simulink model "week4_4_final_cruise_control"  (R2025b)
settings: Solver=VariableStepAuto  StartTime=0.0  StopTime=100  MaxStep=0.01  RelTol=1e-3
undefined symbols (not defined in the file): A_front, Cd, Cr, g, m, rho, v0
libraries: slpidlib x1
settings Model: Creator=legob  LastModifiedBy=legob

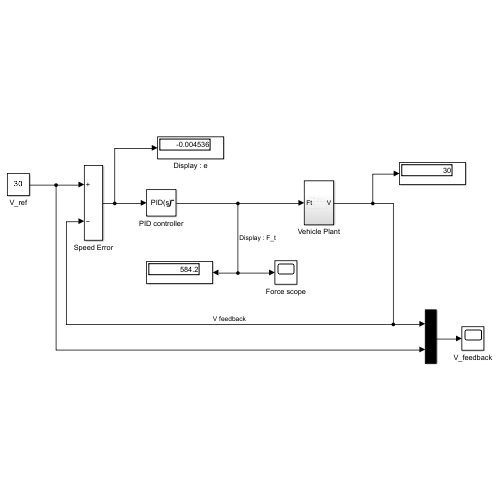
[thumbnail: Simulink's stored preview of the top-level diagram]
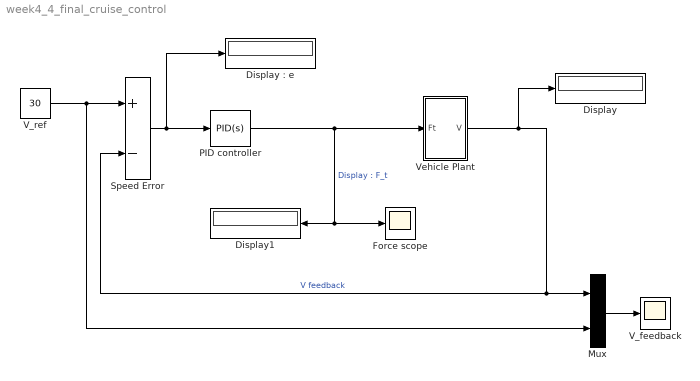
== system week4_4_final_cruise_control ==
  Display : Display
  "Display : e" : Display
  Display1 : Display
  Force scope : Scope
      settings: ActiveDisplayYMinimum=-292.64351118443733  ActiveDisplayYMaximum=5182.92090492779
  Mux : Mux  Inputs=2
  PID controller : slpidlib/PID Controller  Controller=PID  Form=Parallel  TimeDomain=Continuous-time  UseExternalTs=off  SampleTime=-1  IntegratorMethod=Forward Euler  FilterMethod=Forward Euler  ControllerParametersSource=internal  P=500  I=25  UseKiTs=off  D=500  UseExternalDerivativeSource=off  N=100  UseFilter=on  TunerSelectOption=Transfer Function Based (PID Tuner App)  InitialConditionSource=internal  InitialConditionForIntegrator=0  InitialConditionForFilter=0  DifferentiatorICPrevScaledInput=0  ExternalReset=none  TrackingMode=off  Kt=1  LimitOutput=on  SatLimitsSource=internal  UpperSaturationLimit=4000  LowerSaturationLimit=0  LinearizeAsGain=on  AntiWindupMode=clamping  Kb=1  LimitIntegrator=off  UpperIntegratorSaturationLimit=inf  LowerIntegratorSaturationLimit=-inf  POutMin=[]  POutMax=[]  IOutMin=[]  IOutMax=[]  DOutMin=[]  DOutMax=[]  NOutMin=[]  NOutMax=[]  SumOutMin=[]  SumOutMax=[]  SaturationOutMin=[]  SaturationOutMax=[]  PParamMin=[]  PParamMax=[]  IParamMin=[]  IParamMax=[]  DParamMin=[]  DParamMax=[]  NParamMin=[]  NParamMax=[]  KbParamMin=[]  KbParamMax=[]  KtParamMin=[]  KtParamMax=[]  KbOutMin=[]  KbOutMax=[]  KtOutMin=[]  KtOutMax=[]  IntegratorOutMin=[]  IntegratorOutMax=[]  FilterOutMin=[]  FilterOutMax=[]  SumI1OutMin=[]  SumI1OutMax=[]  SumI2OutMin=[]  SumI2OutMax=[]  SumI3OutMin=[]  SumI3OutMax=[]  SumI4OutMin=[]  SumI4OutMax=[]  SumDOutMin=[]  SumDOutMax=[]  DifferentiatorOutMin=[]  DifferentiatorOutMax=[]  FilterDiffOutCoefMin=[]  FilterDiffOutCoefMax=[]  ReciprocalOutMin=[]  ReciprocalOutMax=[]  SumDenOutMin=[]  SumDenOutMax=[]  SumNumOutMin=[]  SumNumOutMax=[]  DivideOutMin=[]  DivideOutMax=[]  UdiffTsProdOutMin=[]  UdiffTsProdOutMax=[]  NTsProdOutMin=[]  NTsProdOutMax=[]  UintegralTsProdOutMin=[]  UintegralTsProdOutMax=[]  UngainTsProdOutMin=[]  UngainTsProdOutMax=[]  ClampingZeroOutDataTypeStr=Inherit: Inherit via back propagation  ClampingZeroOutMin=[]  ClampingZeroOutMax=[]  FilterDenConstantOutDataTypeStr=Inherit: Inherit via back propagation  FilterDenConstantOutMin=[]  FilterDenConstantOutMax=[]  PCopyOutDataTypeStr=Inherit: Inherit via back propagation  PCopyOutMin=[]  PCopyOutMax=[]  NCopyOutDataTypeStr=Inherit: Inherit via back propagation  NCopyOutMin=[]  NCopyOutMax=[]  IntegratorContinuousStateAttributes=''  IntegratorStateMustResolveToSignalObject=off  IntegratorRTWStateStorageClass=Auto  FilterContinuousStateAttributes=''  FilterStateMustResolveToSignalObject=off  FilterRTWStateStorageClass=Auto  ParallelPVariant=InternalParameters  IdealPVariant=Disabled  IVariant=InternalParameters  DVariant=InternalParameters  IntegratorVariant=Continuous  SatVariant=Enabled  AWVariant=ContClampingParallel  PCopyVariant=Disabled  TRVariant=Disabled  FdbkBlocksVariant=Forward  IdealPFdbkVariant=Disabled  SatFdbkVariant=Disabled  DerivativeFilterVariant=ContFilter  NVariant=InternalParameters  NCopyVariant=Disabled  FilterICVariant=InternalICsFilter  IntegratorICVariant=InternalICs  ExternalResetVariant=Disabled  TRSumVariant=Passthrough  SumFdbkVariant=Disabled  SumVariant=Sum_PID  TsampFilterVariant=InternalTs  TsampNgainVariant=Passthrough  TsampIntegralVariant=Disabled_SignalSpec  ExternalSaturationOutDataTypeStr=Inherit: Same as second input  DerivativeSourceVariant=ErrorSignal  PreIntVariant=InternalPreInt
  Speed Error : Sum  Inputs=+-
  V_feedback : Scope
      settings: ActiveDisplayYMinimum=6.99310501020965  ActiveDisplayYMaximum=55.696887760610466
  V_ref : Constant  Value=30
  Vehicle Plant : Subsystem
  wires:
  Vehicle Plant/1(V) -> Speed Error/2, Mux/1, Display/1  "V feedback"
  V_ref/1 -> Mux/2, Speed Error/1
  Speed Error/1 -> "Display : e"/1, PID controller/1
  PID controller/1 -> Force scope/1, Display1/1, Vehicle Plant/1(Ft)  "Display : F_t"
  Mux/1 -> V_feedback/1

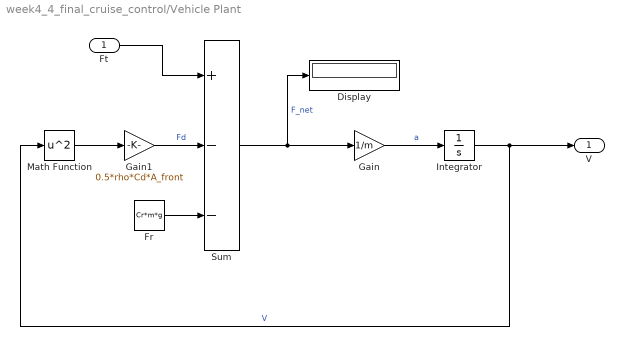
== system week4_4_final_cruise_control/Vehicle Plant ==
  Ft : Inport
  Display : Display
  Fr : Constant  Value=Cr*m*g
  Gain : Gain  Gain=1/m
  Gain1 : Gain  Gain=0.5*rho*Cd*A_front
  Integrator : Integrator  InitialCondition=v0
  Math Function : Math  Operator=square
  Sum : Sum  Inputs=+--
  V : Outport
  wires:
  Fr/1 -> Sum/3
  Integrator/1 -> V/1, Math Function/1  "V"
  Sum/1 -> Display/1, Gain/1  "F_net"
  Gain/1 -> Integrator/1  "a"
  Ft/1 -> Sum/1
  Gain1/1 -> Sum/2  "Fd"
  Math Function/1 -> Gain1/1
